simulink model "openloopFEScontrollerSim"  (R2020b)
settings: Solver=VariableStepAuto  StartTime=0.0  StopTime=100000  RelTol=1e-3
values from neighbouring files (symbols this model uses):
  h_mdls = calibration(elecArray, maxStimAmp, maxForce,h_mdl_struct, bt)    [FES_open_loop.m]
libraries: slident x3, dspnetwork x3, sldrtlib x1
settings Model: Creator=ayurkewi  LastModifiedBy=julie
settings DataIOCC: ReturnWorkspaceOutputs=off
settings DebuggingCC: ArithmeticOperatorsInVariantConditions=warning
settings SFSimCC: CustomCodeUndefinedFunction=UseInterfaceOnly

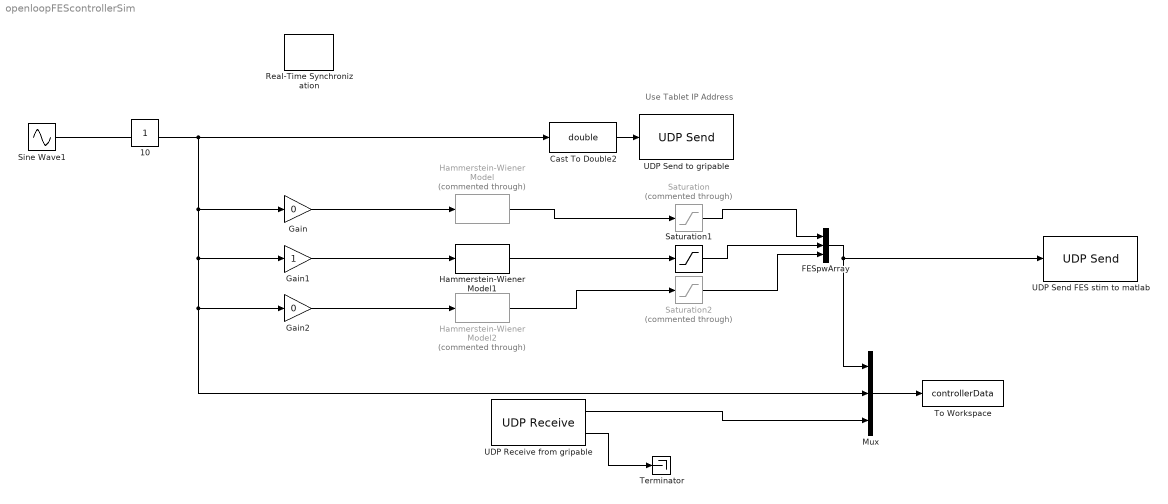
== system openloopFEScontrollerSim ==
  note: Use Tablet IP Address
  Cast To Double2 : DataTypeConversion  OutDataTypeStr=double
  FESpwArray : Mux  Inputs=3
  Gain : Gain  Gain=0
  Gain1 : Gain
  Gain2 : Gain  Gain=0
  Hammerstein-Wiener Model : slident/Models/Hammerstein-Wiener Model  Commented=through  sys=h_mdls{1}  IC=Zero  X0i=0
      settings: SourceProductBaseCode=ID
  Hammerstein-Wiener Model1 : slident/Models/Hammerstein-Wiener Model  sys=h_mdls{1}  IC=Zero  X0i=0
      settings: SourceProductBaseCode=ID
  Hammerstein-Wiener Model2 : slident/Models/Hammerstein-Wiener Model  Commented=through  sys=h_mdls{1}  IC=Zero  X0i=0
      settings: SourceProductBaseCode=ID
  Mux : Mux  Inputs=3
  Real-Time Synchronization : sldrtlib/Real-Time Synchronization  SampleTime=0.001  MaxMissedTicks=100000  ShowMissedTicks=off  YieldWhenWaiting=off
  Saturation : Saturate  Commented=through  UpperLimit=400  LowerLimit=100
  Saturation1 : Saturate  UpperLimit=400  LowerLimit=100
  Saturation2 : Saturate  Commented=through  UpperLimit=400  LowerLimit=100
  Sine Wave1 : Sin  Amplitude=0.03  Bias=0.04  Frequency=0.1  Phase=3/2 *pi  SampleTime=0
  Terminator : Terminator
  To Workspace : ToWorkspace  VariableName=controllerData  SaveFormat=Timeseries  SampleTime=-1
  UDP Receive from gripable : dspnetwork/UDP Receive  localURL='0.0.0.0'  localPort=26000  remoteURL='0.0.0.0'  remotePort=-1  recvBufferSize=8192  dims=1  signalDatatype=double  isComplex=off  isVarSize=off  showBlockingTime=off  blockingTime=0  sampletime=0.001  blockPlatform=[]
  UDP Send FES stim to matlab : dspnetwork/UDP Send  remoteURL='127.0.0.1'  remotePort=22392  localURL='0.0.0.0'  localPortSource=Automatically determine  localPort=-1  sendBufferSize=8192  sampletime=-1  blockPlatform=[]  separateLengthPort=0
  UDP Send to gripable : dspnetwork/UDP Send  remoteURL='146.169.201.205'  remotePort=25000  localURL='0.0.0.0'  localPortSource=Automatically determine  localPort=-1  sendBufferSize=8192  sampletime=-1  blockPlatform=[]  separateLengthPort=0
  10 : Constant  IOType=siggen
  wires:
  Cast To Double2/1 -> UDP Send to gripable/1
  Sine Wave1/1 -> Mux/2, Gain2/1, Gain1/1, Gain/1, Cast To Double2/1
  Hammerstein-Wiener Model/1 -> Saturation/1
  Hammerstein-Wiener Model1/1 -> Saturation1/1
  FESpwArray/1 -> Mux/1, UDP Send FES stim to matlab/1
  Gain/1 -> Hammerstein-Wiener Model/1
  Gain2/1 -> Hammerstein-Wiener Model2/1
  Gain1/1 -> Hammerstein-Wiener Model1/1
  UDP Receive from gripable/2 -> Terminator/1
  UDP Receive from gripable/1 -> Mux/3
  Mux/1 -> To Workspace/1
  Hammerstein-Wiener Model2/1 -> Saturation2/1
  Saturation1/1 -> FESpwArray/2
  Saturation/1 -> FESpwArray/1
  Saturation2/1 -> FESpwArray/3
